simulink model "Tekercs"  (R2025a)
settings: Solver=VariableStepAuto  StartTime=0.0  StopTime=10e-3  MaxStep=20e-6  RelTol=1e-3
settings Model: Creator=Szalay  LastModifiedBy=Szalay

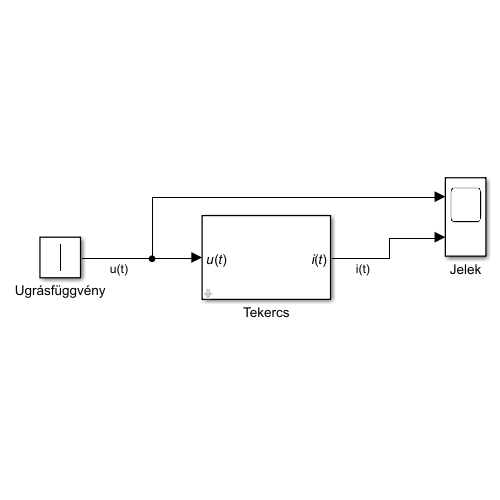
[thumbnail: Simulink's stored preview of the top-level diagram]
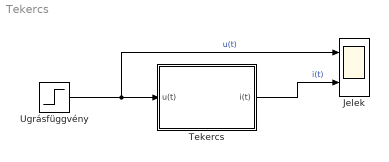
== system Tekercs ==
  Jelek : Scope  NumInputPorts=2
      settings: ActiveDisplayYMinimum=-1.375  ActiveDisplayYMaximum=2.375
  Tekercs : Subsystem  mask(Tekercs){R=1, L=1e-3, i_0=-1}
      mask prompts: R "Ellenállás"; L "Induktivitás"; i_0 "Kezdeti áramerősség"
      mask help: Lineáris mágnesezésű tekercsmodell.
      mask DialogControl ParameterGroupVar Prompt: Modellparaméterek
      mask DialogControl Container3 Prompt: Kezdeti érték
      mask Display:
      | % Csatlakozók
      | port_label('input', 1, '{\itu}({\itt})', 'texmode', 'on');
      | port_label('output', 1, '{\iti}({\itt})', 'texmode', 'on');
  Ugrásfüggvény : Step  Time=1e-3  After=2  SampleTime=0
  wires:
  Ugrásfüggvény/1 -> Jelek/1, Tekercs/1(u(t))  "u(t)"
  Tekercs/1(i(t)) -> Jelek/2  "i(t)"

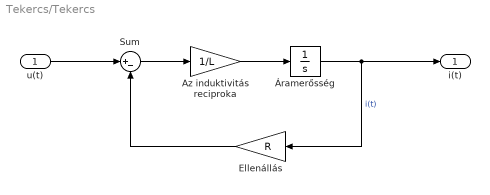
== system Tekercs/Tekercs ==
  u(t) : Inport
  Az induktivitás reciproka : Gain  Gain=1/L
  Ellenállás : Gain  Gain=R
  Sum : Sum  Inputs=|+-
  Áramerősség : Integrator  InitialCondition=i_0
  i(t) : Outport
  wires:
  Az induktivitás reciproka/1 -> Áramerősség/1
  Áramerősség/1 -> i(t)/1, Ellenállás/1  "i(t)"
  Sum/1 -> Az induktivitás reciproka/1
  Ellenállás/1 -> Sum/2
  u(t)/1 -> Sum/1
